simulink model "Synch_Gen7"  (Simulink 4.00)
settings: Solver=ode45  StartTime=0.0  StopTime=10.0  RelTol=1e-3
InitFcn:
  | powericon('psbinitsys',bdroot);
libraries: powerlib2 x11, powerlib11 x2
settings Model: LastModifiedBy=ieao

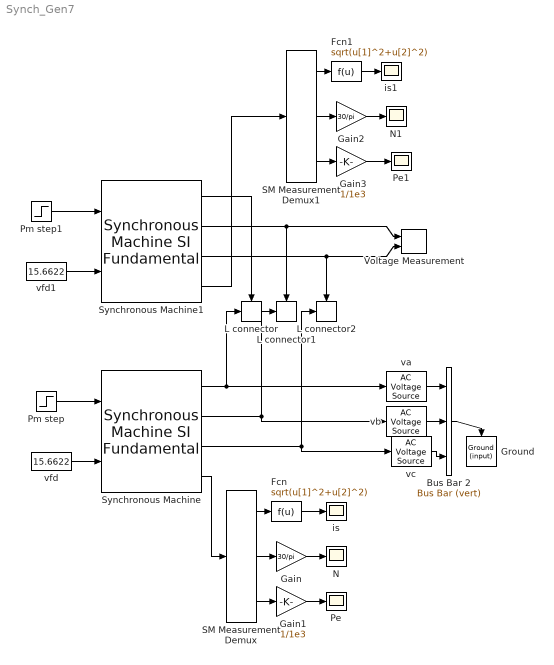
== system Synch_Gen7 ==
  Bus Bar 2 : powerlib2/Connectors/Bus Bar (vert)  Tag=PoWeRsYsTeMbLoCk  entrees=3  sorties=1  PSBOutputType=11111111111111111111111111111111111111111111111111111111111111111111111111111111111111111
  Fcn : Fcn  Expr=sqrt(u[1]^2+u[2]^2)
  Fcn1 : Fcn  Expr=sqrt(u[1]^2+u[2]^2)
  Gain : Gain  Gain=30/pi  Multiplication=Element-wise(K.*u)  SaturateOnIntegerOverflow=on
  Gain1 : Gain  Gain=1/1e3  Multiplication=Element-wise(K.*u)  SaturateOnIntegerOverflow=on
  Gain2 : Gain  Gain=30/pi  Multiplication=Element-wise(K.*u)  SaturateOnIntegerOverflow=on
  Gain3 : Gain  Gain=1/1e3  Multiplication=Element-wise(K.*u)  SaturateOnIntegerOverflow=on
  Ground : powerlib2/Connectors/Ground (input)  Tag=PoWeRsYsTeMbLoCk  Orientation=down
  L connector : powerlib2/Connectors/L connector  Tag=PoWeRsYsTeMbLoCk
  L connector1 : powerlib2/Connectors/L connector  Tag=PoWeRsYsTeMbLoCk
  L connector2 : powerlib2/Connectors/L connector  Tag=PoWeRsYsTeMbLoCk
  N : Scope
      settings: TickLabels=on  TimeRange=5  YMin=1798.5  YMax=1800.5  SaveName=N  DataFormat=Array  MaxDataPoints=5000
  N1 : Scope
      settings: TickLabels=on  TimeRange=5  YMin=1798.5  YMax=1800.5  SaveName=N1  DataFormat=Array  MaxDataPoints=5000
  Pe : Scope
      settings: TickLabels=on  TimeRange=5  YMin=-25  YMax=25  SaveName=Pe  DataFormat=Array  MaxDataPoints=5000
  Pe1 : Scope
      settings: TickLabels=on  TimeRange=5  YMin=-35  YMax=35  SaveName=Pe1  DataFormat=Array  MaxDataPoints=5000
  Pm step : Step  Time=0.5  Before=-50000  After=-60000  SampleTime=0
  Pm step1 : Step  Time=0.5  Before=-50000  After=-60000  SampleTime=0
  SM Measurement Demux : powerlib11/Machines/SM Measurement Demux  a=off  b=on  c=off  d=off  e=off  f=off  g=off  h=on  i=on  j=off
  SM Measurement Demux1 : powerlib11/Machines/SM Measurement Demux  a=off  b=on  c=off  d=off  e=off  f=off  g=off  h=on  i=on  j=off
  Synchronous Machine : powerlib2/Machines/Synchronous Machine SI Fundamental  Tag=PoWeRsYsTeMbLoCk  rotorType=Salient-pole  x1="[ 111900 440*sqrt(3) 60  0]"  x2=[ .26 1.14e-3 13.7e-3 11.0e-3 ]  x3=[ 0.13 2.1e-3 ]  x4b=[ 1 2 3 4 5 6 ]  x4=[ 0.0224 1.4e-3 0.02 1e-3 ]  x5=[ 24.9 0 2 ]  x6="[ 0  335.978  55.9962,55.9962,55.9962  258.5352,138.5352,18.5352  15.6622 ]"  x7=off  x8=[]  x9=off  PSBOutputType=1110  iounits=1
  Synchronous Machine1 : powerlib2/Machines/Synchronous Machine SI Fundamental  Tag=PoWeRsYsTeMbLoCk  rotorType=Salient-pole  x1="[ 111900 440*sqrt(3) 60  0]"  x2=[ .26 1.14e-3 13.7e-3 11.0e-3 ]  x3=[ 0.13 2.1e-3 ]  x4b=[ 1 2 3 4 5 6 ]  x4=[ 0.0224 1.4e-3 0.02 1e-3 ]  x5=[ 24.9 0 2 ]  x6="[ 0  335.978  55.9962,55.9962,55.9962  258.5352,138.5352,18.5352  15.6622 ]"  x7=off  x8=[]  x9=off  PSBOutputType=1110  iounits=1
  Voltage Measurement : powerlib2/Measurements/Voltage Measurement  Tag=PoWeRsYsTeMmEaSuReMeNt  PSBOutputType=0  PSBequivalent=1
  is : Scope
      settings: TickLabels=on  TimeRange=5  YMin=55  YMax=75  SaveName=is  DataFormat=Array  MaxDataPoints=5000
  is1 : Scope
      settings: TickLabels=on  TimeRange=5  YMin=55  YMax=75  SaveName=is1  DataFormat=Array  MaxDataPoints=5000
  va : powerlib2/Electrical Sources/AC Voltage Source  Tag=PoWeRsYsTeMbLoCk  A=440*sqrt(2)  P=270  F=60  stime=0  mesure=None  PSBOutputType=1
  vb : powerlib2/Electrical Sources/AC Voltage Source  Tag=PoWeRsYsTeMbLoCk  A=440*sqrt(2)  P=150  F=60  stime=0  mesure=None  PSBOutputType=1
  vc : powerlib2/Electrical Sources/AC Voltage Source  Tag=PoWeRsYsTeMbLoCk  A=440*sqrt(2)  P=30  F=60  stime=0  mesure=None  PSBOutputType=1
  vfd : Constant  Value=15.6622
  vfd1 : Constant  Value=15.6622
  wires:
  Synchronous Machine/4 -> SM Measurement Demux/1
  vfd/1 -> Synchronous Machine/2
  va/1 -> Bus Bar 2/1
  vb/1 -> Bus Bar 2/2
  vc/1 -> Bus Bar 2/3
  Pm step/1 -> Synchronous Machine/1
  Fcn/1 -> is/1
  SM Measurement Demux/1 -> Fcn/1
  SM Measurement Demux/2 -> Gain/1
  SM Measurement Demux/3 -> Gain1/1
  Gain/1 -> N/1
  Gain1/1 -> Pe/1
  vfd1/1 -> Synchronous Machine1/2
  Pm step1/1 -> Synchronous Machine1/1
  Synchronous Machine1/1 -> L connector/Enable
  Synchronous Machine1/2 -> L connector1/Enable, Voltage Measurement/1
  Synchronous Machine1/3 -> L connector2/Enable, Voltage Measurement/2
  Synchronous Machine/1 -> L connector/1, va/1
  Synchronous Machine/2 -> L connector1/1, vb/1
  Synchronous Machine/3 -> L connector2/1, vc/1
  Bus Bar 2/1 -> Ground/1
  Fcn1/1 -> is1/1
  SM Measurement Demux1/1 -> Fcn1/1
  SM Measurement Demux1/2 -> Gain2/1
  SM Measurement Demux1/3 -> Gain3/1
  Gain2/1 -> N1/1
  Gain3/1 -> Pe1/1
  Synchronous Machine1/4 -> SM Measurement Demux1/1
